simulink subsystem "ideal_pistons"  (R2022b)
settings: Solver=VariableStepAuto  StartTime=0.0  StopTime=10.0  RelTol=1e-3
values from neighbouring files (symbols this model uses):
  displacer_piston = struct()    [Large_engine_params.m]    (also in Small_engine_params.m)
libraries: fl_lib x17, nesl_utility x4
settings Model: Creator=wilde  LastModifiedBy=wilde

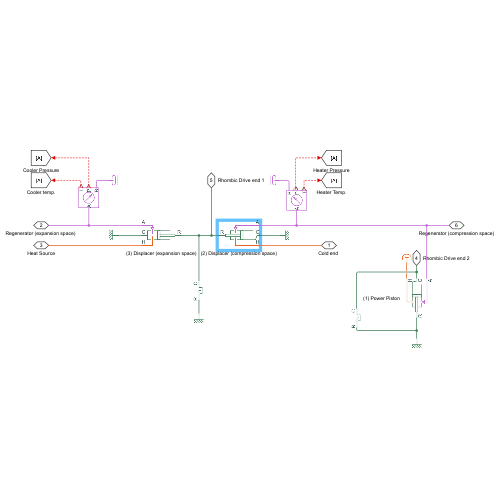
[thumbnail: Simulink's stored preview of the top-level diagram]
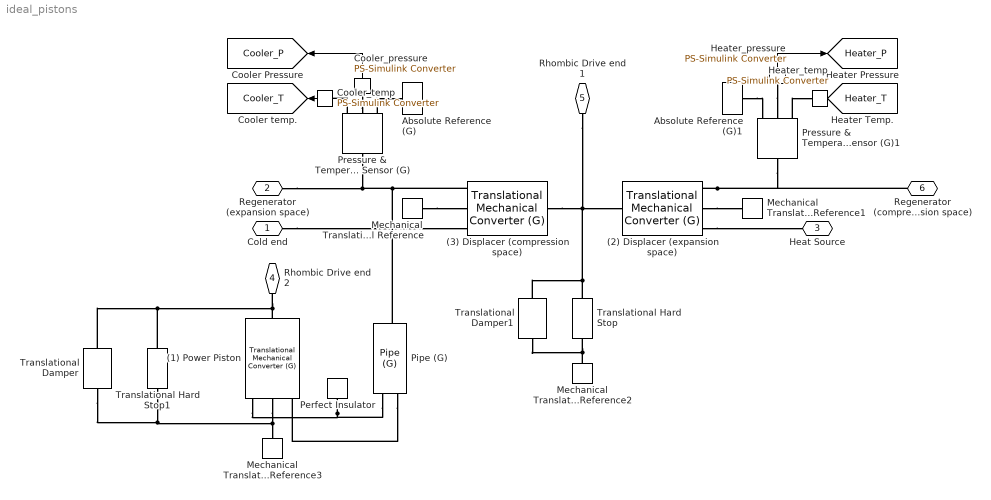
== system ideal_pistons ==
  (1) Power Piston : fl_lib/Gas/Elements/Translational Mechanical Converter (G)  mech_orientation=foundation.enum.MechOrientationTranslational.Negative  displacement_spec=foundation.enum.DisplacementSpec.Calculate  length_init=power_piston.piston.ini_disp m  interface_area=power_piston.piston.interf_area m^2  dead_volume=power_piston.piston.dead_vol m^3  area_A=passage_pipe.geom.area m^2  environment_spec=foundation.enum.pressure_spec.specified  environment_pressure=ambient.pext MPa  p_I_specify=on  p_I_priority=High  p_I=state_init.p0 MPa  p_I_nominal_specify=off  p_I_nominal_unit=MPa  p_I_nominal_value=1  T_I_specify=on  T_I_priority=High  T_I=ambient.temperature K  T_I_nominal_specify=off  T_I_nominal_unit=K  T_I_nominal_value=1  rho_converter_specify=off  rho_converter_priority=None  rho_converter=1.2 kg/m^3  rho_converter_nominal_specify=off  rho_converter_nominal_unit=kg/m^3  rho_converter_nominal_value=1.6
      settings: InternalSimscapePortConfiguration="{\"Bottom\":[],\"Left\":[{\"id\":\"A\",\"label\":\"A\",\"type\":\"foundation.gas.gas\"},{\"id\":\"C\",\"label\":\"C\",\"type\":\"foundation.mechanical.translational.translational\"},{\"id\":\"H\",\"label\":\"H\",\"type\":\"foundation.thermal.thermal\"}],\"Right\":[{\"id\":\"R\",\"label\":\"R\",\"type\":\"foundation.mechanical.translational.translational\"}],\"Top\":[]}"
  (2) Displacer (expansion space) : fl_lib/Gas/Elements/Translational Mechanical Converter (G)  mech_orientation=foundation.enum.MechOrientationTranslational.Negative  displacement_spec=foundation.enum.DisplacementSpec.Calculate  length_init=displacer_piston.piston.ini_disp_heater m  interface_area=displacer_piston.piston.interf_area m^2  dead_volume=displacer_piston.piston.dead_vol m^3  area_A=displacer_piston.piston.portA_area m^2  environment_spec=foundation.enum.pressure_spec.specified  environment_pressure=ambient.pext MPa  p_I_specify=on  p_I_priority=High  p_I=state_init.p0 MPa  p_I_nominal_specify=off  p_I_nominal_unit=MPa  p_I_nominal_value=1  T_I_specify=on  T_I_priority=High  T_I=state_init.T0 K  T_I_nominal_specify=off  T_I_nominal_unit=K  T_I_nominal_value=1  rho_converter_specify=off  rho_converter_priority=None  rho_converter=1.2 kg/m^3  rho_converter_nominal_specify=off  rho_converter_nominal_unit=kg/m^3  rho_converter_nominal_value=1.6
      settings: InternalSimscapePortConfiguration="{\"Bottom\":[],\"Left\":[{\"id\":\"A\",\"label\":\"A\",\"type\":\"foundation.gas.gas\"},{\"id\":\"C\",\"label\":\"C\",\"type\":\"foundation.mechanical.translational.translational\"},{\"id\":\"H\",\"label\":\"H\",\"type\":\"foundation.thermal.thermal\"}],\"Right\":[{\"id\":\"R\",\"label\":\"R\",\"type\":\"foundation.mechanical.translational.translational\"}],\"Top\":[]}"
  (3) Displacer (compression space) : fl_lib/Gas/Elements/Translational Mechanical Converter (G)  mech_orientation=foundation.enum.MechOrientationTranslational.Positive  displacement_spec=foundation.enum.DisplacementSpec.Calculate  length_init=displacer_piston.piston.ini_disp_cooler m  interface_area=displacer_piston.piston.interf_area m^2  dead_volume=displacer_piston.piston.dead_vol m^3  area_A=displacer_piston.piston.portA_area m^2  environment_spec=foundation.enum.pressure_spec.specified  environment_pressure=ambient.pext MPa  p_I_specify=on  p_I_priority=High  p_I=state_init.p0 MPa  p_I_nominal_specify=off  p_I_nominal_unit=MPa  p_I_nominal_value=1  T_I_specify=on  T_I_priority=High  T_I=ambient.temperature K  T_I_nominal_specify=off  T_I_nominal_unit=K  T_I_nominal_value=1  rho_converter_specify=off  rho_converter_priority=None  rho_converter=1.2 kg/m^3  rho_converter_nominal_specify=off  rho_converter_nominal_unit=kg/m^3  rho_converter_nominal_value=1.6
      settings: InternalSimscapePortConfiguration="{\"Bottom\":[],\"Left\":[{\"id\":\"A\",\"label\":\"A\",\"type\":\"foundation.gas.gas\"},{\"id\":\"C\",\"label\":\"C\",\"type\":\"foundation.mechanical.translational.translational\"},{\"id\":\"H\",\"label\":\"H\",\"type\":\"foundation.thermal.thermal\"}],\"Right\":[{\"id\":\"R\",\"label\":\"R\",\"type\":\"foundation.mechanical.translational.translational\"}],\"Top\":[]}"
  Absolute Reference (G) : fl_lib/Gas/Elements/Absolute Reference (G)
      settings: InternalSimscapePortConfiguration="{\"Bottom\":[],\"Left\":[{\"id\":\"A\",\"label\":\"\",\"type\":\"foundation.gas.gas\"}],\"Right\":[],\"Top\":[]}"
  Absolute Reference (G)1 : fl_lib/Gas/Elements/Absolute Reference (G)
      settings: InternalSimscapePortConfiguration="{\"Bottom\":[],\"Left\":[{\"id\":\"A\",\"label\":\"\",\"type\":\"foundation.gas.gas\"}],\"Right\":[],\"Top\":[]}"
  Cooler_pressure : nesl_utility/PS-Simulink Converter  PhysicalDomain=network_engine_domain  SubClassName=ps_output  LeftPortType=input  RightPortType=output  PseudoPeriodic=off  Frequencies=[]  VectorFormat=inherit  Unit=inherit  AffineConversion=off
  Cooler_temp : nesl_utility/PS-Simulink Converter  PhysicalDomain=network_engine_domain  SubClassName=ps_output  LeftPortType=input  RightPortType=output  PseudoPeriodic=off  Frequencies=[]  VectorFormat=inherit  Unit=inherit  AffineConversion=off
  Heater_pressure : nesl_utility/PS-Simulink Converter  PhysicalDomain=network_engine_domain  SubClassName=ps_output  LeftPortType=input  RightPortType=output  PseudoPeriodic=off  Frequencies=[]  VectorFormat=inherit  Unit=inherit  AffineConversion=off
  Heater_temp : nesl_utility/PS-Simulink Converter  PhysicalDomain=network_engine_domain  SubClassName=ps_output  LeftPortType=input  RightPortType=output  PseudoPeriodic=off  Frequencies=[]  VectorFormat=inherit  Unit=inherit  AffineConversion=off
  Mechanical Translational Reference{,1..3} (4 alike) : fl_lib/Mechanical/Translational Elements/Mechanical Translational Reference
  Perfect Insulator : fl_lib/Thermal/Thermal Elements/Perfect Insulator  T_specify=off  T_priority=None  T=293.15 K  T_nominal_specify=off  T_nominal_unit=K  T_nominal_value=1
  Pipe (G) : fl_lib/Gas/Elements/Pipe (G)  length=passage_pipe.geom.length m  area=passage_pipe.geom.area m^2  Dh=passage_pipe.geom.hydraulic_diam m  length_add=passage_pipe.therm_fric.length_add m  roughness=passage_pipe.therm_fric.roughness m  Re_lam=passage_pipe.therm_fric.Re_lam  Re_tur=passage_pipe.therm_fric.Re_tur  shape_factor=passage_pipe.therm_fric.shape_factor  Nu_lam=passage_pipe.therm_fric.Nu_lam  p_I_specify=on  p_I_priority=High  p_I=state_init.p0 MPa  p_I_nominal_specify=off  p_I_nominal_unit=MPa  p_I_nominal_value=1  T_I_specify=on  T_I_priority=High  T_I=state_init.T0 K  T_I_nominal_specify=off  T_I_nominal_unit=K  T_I_nominal_value=1  rho_pipe_specify=off  rho_pipe_priority=None  rho_pipe=1.2 kg/m^3  rho_pipe_nominal_specify=off  rho_pipe_nominal_unit=kg/m^3  rho_pipe_nominal_value=1
  Pressure & Temperature Sensor (G) : fl_lib/Gas/Sensors/Pressure & Temperature Sensor (G)
      settings: InternalSimscapePortConfiguration="{\"Bottom\":[],\"Left\":[{\"id\":\"A\",\"label\":\"A\",\"type\":\"foundation.gas.gas\"}],\"Right\":[{\"id\":\"B\",\"label\":\"B\",\"type\":\"foundation.gas.gas\"},{\"id\":\"P\",\"label\":\"P\",\"type\":\"output\"},{\"id\":\"T\",\"label\":\"T\",\"type\":\"output\"}],\"Top\":[]}"
  Pressure & Temperature Sensor (G)1 : fl_lib/Gas/Sensors/Pressure & Temperature Sensor (G)
      settings: InternalSimscapePortConfiguration="{\"Bottom\":[],\"Left\":[{\"id\":\"A\",\"label\":\"A\",\"type\":\"foundation.gas.gas\"}],\"Right\":[{\"id\":\"B\",\"label\":\"B\",\"type\":\"foundation.gas.gas\"},{\"id\":\"P\",\"label\":\"P\",\"type\":\"output\"},{\"id\":\"T\",\"label\":\"T\",\"type\":\"output\"}],\"Top\":[]}"
  Translational Damper : fl_lib/Mechanical/Translational Elements/Translational Damper  D=0.0001 N*s/m  v_specify=off  v_priority=None  v=0 m/s  v_nominal_specify=off  v_nominal_unit=m/s  v_nominal_value=1  f_specify=off  f_priority=None  f=0 N  f_nominal_specify=off  f_nominal_unit=N  f_nominal_value=1
  Translational Damper1 : fl_lib/Mechanical/Translational Elements/Translational Damper  D=0.0001 N*s/m  v_specify=off  v_priority=None  v=0 m/s  v_nominal_specify=off  v_nominal_unit=m/s  v_nominal_value=1  f_specify=off  f_priority=None  f=0 N  f_nominal_specify=off  f_nominal_unit=N  f_nominal_value=1
  Translational Hard Stop : fl_lib/Mechanical/Translational Elements/Translational Hard Stop  upper_bnd=displacer_piston.hardstop.upbound m  lower_bnd=displacer_piston.hardstop.lowbound m  stiff_up=1e10 N/m  stiff_low=1e10 N/m  D_up=1e5 N*s/m  D_low=1e5 N*s/m  model=simscape.enum.hardstop.smooth  transition=displacer_piston.hardstop.trans_region mm  v_specify=off  v_priority=None  v=0 m/s  v_nominal_specify=off  v_nominal_unit=m/s  v_nominal_value=1  f_specify=off  f_priority=None  f=0 N  f_nominal_specify=off  f_nominal_unit=N  f_nominal_value=1  x_specify=on  x_priority=High  x=max(displacer_piston.piston.ini_disp_cooler) m  x_nominal_specify=off  x_nominal_unit=m  x_nominal_value=1
  Translational Hard Stop1 : fl_lib/Mechanical/Translational Elements/Translational Hard Stop  upper_bnd=power_piston.hardstop.upbound m  lower_bnd=power_piston.hardstop.lowbound m  stiff_up=1e7 N/m  stiff_low=1e7 N/m  D_up=1e3 N*s/m  D_low=1e3 N*s/m  model=simscape.enum.hardstop.smooth  transition=displacer_piston.hardstop.trans_region mm  v_specify=off  v_priority=None  v=0 m/s  v_nominal_specify=off  v_nominal_unit=m/s  v_nominal_value=1  f_specify=off  f_priority=None  f=0 N  f_nominal_specify=off  f_nominal_unit=N  f_nominal_value=1  x_specify=on  x_priority=High  x=power_piston.piston.ini_disp m  x_nominal_specify=off  x_nominal_unit=m  x_nominal_value=1
  "Cold end " : PMIOPort  Side=Left
  "Regenerator (expansion space) " : PMIOPort  Port=2  Side=Left
  Heat Source : PMIOPort  Port=3  Side=Right
  Rhombic Drive end 2 : PMIOPort  Port=4  Side=Right
  Rhombic Drive end 1 : PMIOPort  Port=5  Side=Left
  Regenerator (compression space) : PMIOPort  Port=6  Side=Right
  tag scope: Cooler_P=global, Cooler_T=global, Heater_P=global, Heater_T=global
  wires:
  Heater_temp/1 -> [Heater_T]
  Cooler_pressure/1 -> [Cooler_P]
  Cooler_temp/1 -> [Cooler_T]
  Heater_pressure/1 -> [Heater_P]
  connections:
  (2) Displacer (expansion space)/LConn1 -- Pressure & Temperature Sensor (G)1/LConn1 -- Regenerator (compression space)/RConn1
  Pipe (G)/RConn1 -- Pressure & Temperature Sensor (G)/LConn1 -- "Regenerator (expansion space) "/RConn1 -- (3) Displacer (compression space)/LConn1
  Translational Hard Stop/RConn1 -- (2) Displacer (expansion space)/RConn1 -- (3) Displacer (compression space)/RConn1 -- Rhombic Drive end 1/RConn1 -- Translational Damper1/LConn1
  Translational Hard Stop1/LConn1 -- Mechanical Translational Reference3/LConn1 -- (1) Power Piston/LConn2 -- Translational Damper/RConn1
  Translational Hard Stop1/RConn1 -- Rhombic Drive end 2/RConn1 -- (1) Power Piston/RConn1 -- Translational Damper/LConn1
  Perfect Insulator/LConn1 -- (1) Power Piston/LConn3 -- Pipe (G)/LConn2
  Mechanical Translational Reference2/LConn1 -- Translational Hard Stop/LConn1 -- Translational Damper1/RConn1
  (2) Displacer (expansion space)/LConn2 -- Mechanical Translational Reference1/LConn1
  Absolute Reference (G)1/LConn1 -- Pressure & Temperature Sensor (G)1/RConn1
  Pressure & Temperature Sensor (G)/RConn1 -- Absolute Reference (G)/LConn1
  Mechanical Translational Reference/LConn1 -- (3) Displacer (compression space)/LConn2
  Cooler_pressure/LConn1 -- Pressure & Temperature Sensor (G)/RConn2
  Pressure & Temperature Sensor (G)/RConn3 -- Cooler_temp/LConn1
  Pressure & Temperature Sensor (G)1/RConn3 -- Heater_temp/LConn1
  Heater_pressure/LConn1 -- Pressure & Temperature Sensor (G)1/RConn2
  (2) Displacer (expansion space)/LConn3 -- Heat Source/RConn1
  "Cold end "/RConn1 -- (3) Displacer (compression space)/LConn3
  Pipe (G)/LConn1 -- (1) Power Piston/LConn1
